simulink library "rudderController"  (R2018a)
settings: Solver=VariableStepAuto  StartTime=0.0  StopTime=10.0  RelTol=1e-3
undefined symbols (not defined in the file): iterationPhase_enum
libraries: calculateReelInRudderAngle x1, calculateReelOutRudderAngle x1, simulink x1, saturateRudderAngle x1
settings Model: Creator=mitch  LastModifiedBy=M.Cobb

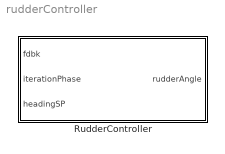
== system rudderController ==
  RudderController : Subsystem

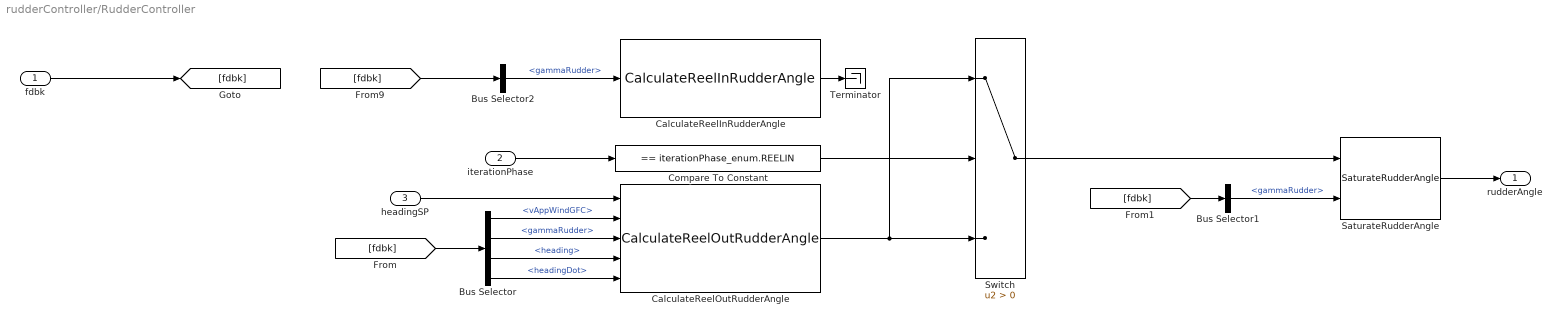
== system rudderController/RudderController ==
  fdbk : Inport  OutDataTypeStr=Bus: busPlantFeedback
  iterationPhase : Inport  Port=2  Unit=rad
  headingSP : Inport  Port=3  Unit=rad
  Bus Selector : BusSelector  OutputSignals=vAppWindGFC,gammaRudder,heading,headingDot
  Bus Selector1 : BusSelector  OutputSignals=gammaRudder
  Bus Selector2 : BusSelector  OutputSignals=gammaRudder
  CalculateReelInRudderAngle : calculateReelInRudderAngle/CalculateReelInRudderAngle
  CalculateReelOutRudderAngle : calculateReelOutRudderAngle/CalculateReelOutRudderAngle
  Compare To Constant : simulink/Logic and Bit Operations/Compare To Constant  relop===  const=iterationPhase_enum.REELIN  OutDataTypeStr=boolean
  "SaturateRudderAngle " : saturateRudderAngle/SaturateRudderAngle 
  Switch : Switch  Criteria=u2 > Threshold
  Terminator : Terminator
  rudderAngle : Outport  Unit=rad
  wires:
  CalculateReelInRudderAngle/1 -> Terminator/1
  "SaturateRudderAngle "/1 -> rudderAngle/1
  CalculateReelOutRudderAngle/1 -> Switch/1, Switch/3
  fdbk/1 -> [fdbk]
  Compare To Constant/1 -> Switch/2
  iterationPhase/1 -> Compare To Constant/1
  Switch/1 -> "SaturateRudderAngle "/1
  Bus Selector1/1 -> "SaturateRudderAngle "/2  "<gammaRudder>"
  [fdbk] -> Bus Selector1/1
  Bus Selector2/1 -> CalculateReelInRudderAngle/1  "<gammaRudder>"
  [fdbk] -> Bus Selector2/1
  [fdbk] -> Bus Selector/1
  headingSP/1 -> CalculateReelOutRudderAngle/1
  Bus Selector/1 -> CalculateReelOutRudderAngle/2  "<vAppWindGFC>"
  Bus Selector/2 -> CalculateReelOutRudderAngle/3  "<gammaRudder>"
  Bus Selector/3 -> CalculateReelOutRudderAngle/4  "<heading>"
  Bus Selector/4 -> CalculateReelOutRudderAngle/5  "<headingDot>"
